simulink model "exnb4137986_Q10"  (R2023b)
settings: Solver=VariableStepAuto  StartTime=0.0  StopTime=10.0  RelTol=1e-3
values from neighbouring files (symbols this model uses):
  A = double(A)    [exnb4137986_Q10_par.m]    (also in exnb4137986_Q5_par.m; exnb4137986_Q7_par.m; exnb4137986_Q8_par.m; exnb4137986_Q9_par.m)
  B = double(diff(X_dot, u))    [exnb4137986_Q10_par.m]    (also in exnb4137986_Q5_par.m; exnb4137986_Q7_par.m; exnb4137986_Q8_par.m; exnb4137986_Q9_par.m)
  C = [0, 1]    [exnb4137986_Q10_par.m]    (also in exnb4137986_Q5_par.m = [C, A^i * B]; exnb4137986_Q7_par.m; exnb4137986_Q8_par.m = [0 1]; exnb4137986_Q9_par.m = jacobian(y, X))
  L = acker(A', C', p_obs_des)'    [exnb4137986_Q10_par.m]
  values = [0, 0.01, 1, 0.001, 1, 1, 10]    [exnb4137986_Q10_par.m]    (also in exnb4137986_Q4_par.m; exnb4137986_Q5_par.m; exnb4137986_Q7_par.m; exnb4137986_Q8_par.m)
  x_star_1 = [I_star_1, omega_star_1]    [exnb4137986_Q10_par.m]    (also in exnb4137986_Q4_par.m = [omega_star_1, I_star_1]; exnb4137986_Q5_par.m; exnb4137986_Q7_par.m; exnb4137986_Q8_par.m)
  x_star_2 = [0, 10]    [exnb4137986_Q10_par.m]    (also in exnb4137986_Q7_par.m; exnb4137986_Q8_par.m)
settings Model: Creator=therkelsen  LastModifiedBy=therkelsen

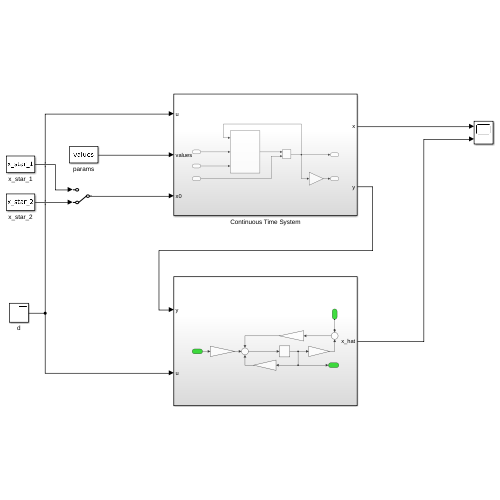
[thumbnail: Simulink's stored preview of the top-level diagram]
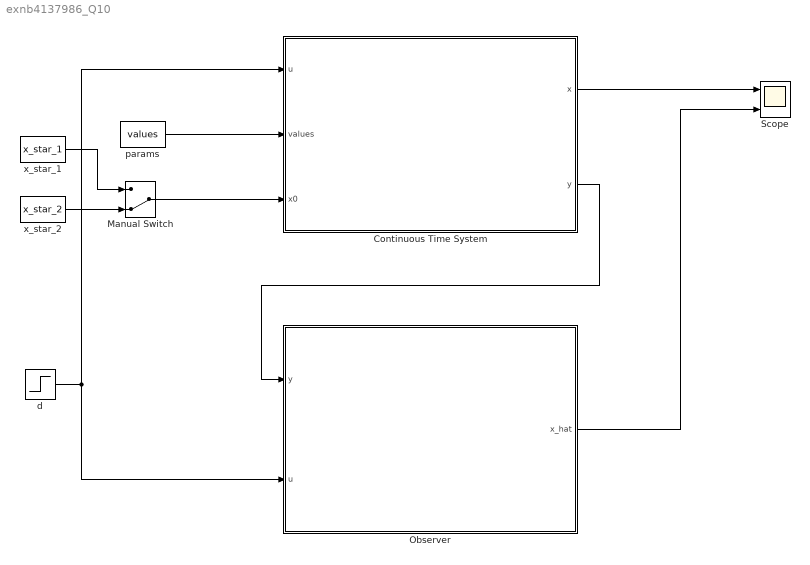
== system exnb4137986_Q10 ==
  Continuous Time System : Subsystem
  Manual Switch : ManualSwitch  CurrentSetting=0
  Observer : Subsystem
  Scope : Scope  NumInputPorts=2
  d : Step  Time=2  After=0  SampleTime=0
  params : Constant  Value=values
  x_star_1 : Constant  Value=x_star_1
  x_star_2 : Constant  Value=x_star_2
  wires:
  Continuous Time System/1(x) -> Scope/1
  params/1 -> Continuous Time System/2(values)
  Manual Switch/1 -> Continuous Time System/3(x0)
  x_star_1/1 -> Manual Switch/1
  x_star_2/1 -> Manual Switch/2
  d/1 -> Continuous Time System/1(u), Observer/2(u)
  Observer/1(x_hat) -> Scope/2
  Continuous Time System/2(y) -> Observer/1(y)

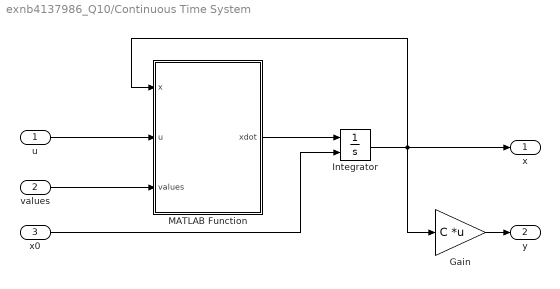
== system exnb4137986_Q10/Continuous Time System ==
  u : Inport
  values : Inport  Port=2
  x0 : Inport  Port=3
  Gain : Gain  Gain=C  Multiplication=Matrix(K*u) (u vector)
  Integrator : Integrator  InitialConditionSource=external
  MATLAB Function : MATLAB Function  TreatAsAtomicUnit=on
  x : Outport
  y : Outport  Port=2
  wires:
  MATLAB Function/1(xdot) -> Integrator/1
  values/1 -> MATLAB Function/3(values)
  u/1 -> MATLAB Function/2(u)
  Integrator/1 -> Gain/1, x/1, MATLAB Function/1(x)
  x0/1 -> Integrator/2
  Gain/1 -> y/1

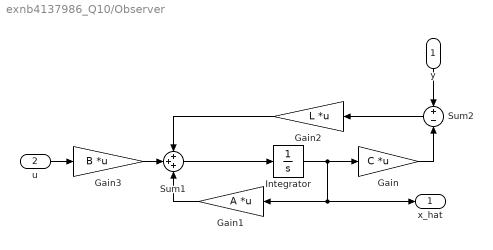
== system exnb4137986_Q10/Observer ==
  y : Inport
  u : Inport  Port=2
  Gain : Gain  Gain=C  Multiplication=Matrix(K*u) (u vector)
  Gain1 : Gain  Gain=A  Multiplication=Matrix(K*u) (u vector)
  Gain2 : Gain  Gain=L  Multiplication=Matrix(K*u) (u vector)
  Gain3 : Gain  Gain=B  Multiplication=Matrix(K*u) (u vector)
  Integrator : Integrator  InitialCondition=[2, -20]
  Sum1 : Sum  Inputs=+++
  Sum2 : Sum  Inputs=+-
  x_hat : Outport
  wires:
  Sum2/1 -> Gain2/1
  Integrator/1 -> Gain1/1, x_hat/1, Gain/1
  y/1 -> Sum2/1
  Gain2/1 -> Sum1/1
  Gain1/1 -> Sum1/3
  Sum1/1 -> Integrator/1
  Gain/1 -> Sum2/2
  Gain3/1 -> Sum1/2
  u/1 -> Gain3/1

== matlab function exnb4137986_Q10/Continuous Time System/MATLAB Function ==
  data: x input; u input; xdot output; values input
function xdot = fcn(x, u, values)

J = values(2);
L = values(3);
Kd = values(4);
Ke = values(5);
Km = values(6);
Rm = values(7);

xdot = [-Rm/L * x(1) - Ke/L * x(2) + 1/L * u;
         Km/J * x(1) - Kd/J * x(2)];
